simulink model "AnalysisSample11"  (R2021b)
settings: Solver=VariableStepAuto  StartTime=0.0  StopTime=10.0  RelTol=1e-3
settings Model: Creator=ygkwon  LastModifiedBy=ygkwon

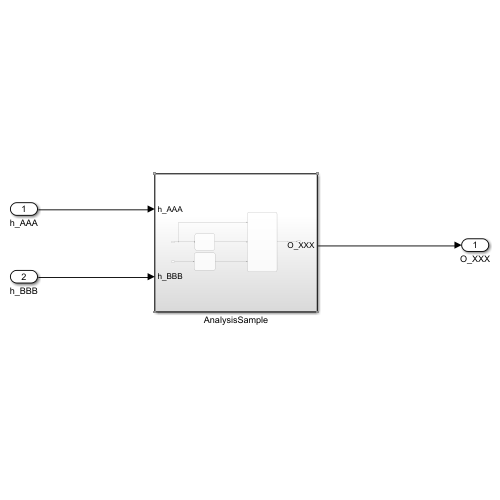
[thumbnail: Simulink's stored preview of the top-level diagram]
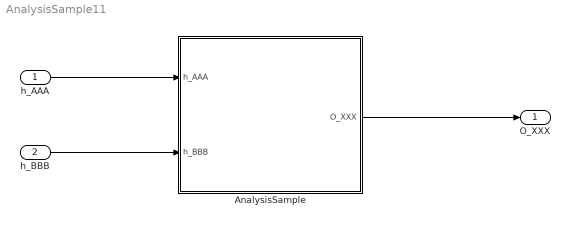
== system AnalysisSample11 ==
  h_AAA : Inport
  h_BBB : Inport  Port=2
  AnalysisSample : Subsystem
  O_XXX : Outport
  wires:
  h_AAA/1 -> AnalysisSample/1(h_AAA)
  AnalysisSample/1(O_XXX) -> O_XXX/1
  h_BBB/1 -> AnalysisSample/2(h_BBB)

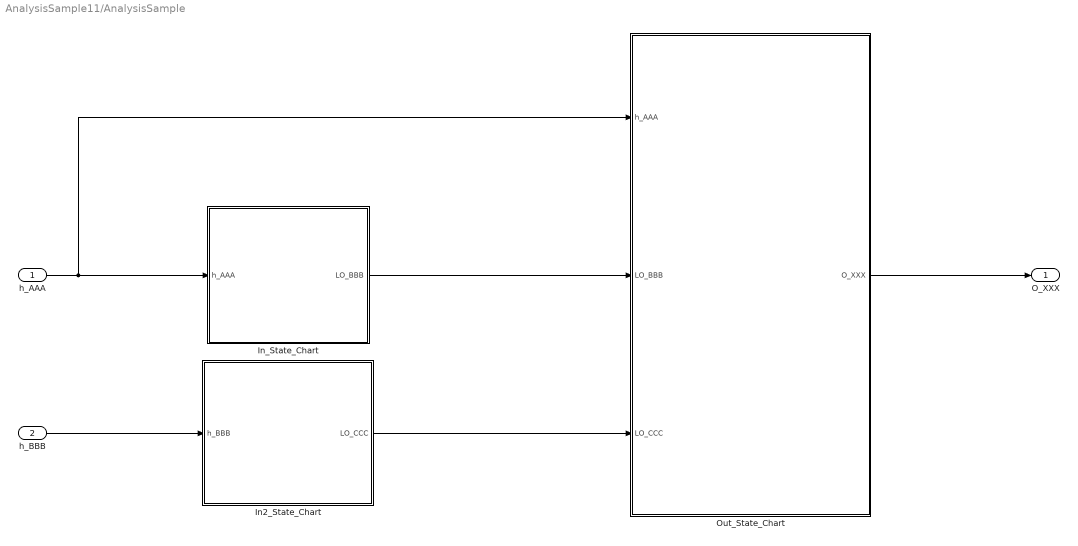
== system AnalysisSample11/AnalysisSample ==
  h_AAA : Inport
  h_BBB : Inport  Port=2
  In2_State_Chart : Stateflow chart  TreatAsAtomicUnit=on
  In_State_Chart : Stateflow chart  TreatAsAtomicUnit=on
  Out_State_Chart : Stateflow chart  TreatAsAtomicUnit=on
  O_XXX : Outport
  wires:
  In_State_Chart/1(LO_BBB) -> Out_State_Chart/2(LO_BBB)
  h_AAA/1 -> Out_State_Chart/1(h_AAA), In_State_Chart/1(h_AAA)
  Out_State_Chart/1(O_XXX) -> O_XXX/1
  h_BBB/1 -> In2_State_Chart/1(h_BBB)
  In2_State_Chart/1(LO_CCC) -> Out_State_Chart/3(LO_CCC)

== stateflow chart AnalysisSample11/AnalysisSample/In_State_Chart ==
  state Sample_State_Chart_2222
    en:
    LO_BBB = 22;
    state a
      en:
      LO_BBB=1;
    state a1
      en:
      LO_BBB=2;
    state a2
      en:
      LO_BBB=1;
    state a3
      en:
      LO_BBB=2;
      du:
      hello();
    (default) -> a [order 1] : [h_AAA == 11]
    a1 -> a [order 1] : [h_AAA==1]
    a1 -> a [order 2] : [h_AAA==11]
    a -> a1 : [h_AAA==2]
    (default) -> a2 [order 2]
    a3 -> a2 [order 1] : [h_AAA==1]
        | %hello
    a3 -> a2 [order 2] : [h_AAA==11]
    a2 -> a3 : [h_AAA==2]
  state hello [function]
    (default) -> (junction 20)
    (junction 20) -> (junction 24) [order 1] : [h_AAA == 111]
    (junction 20) -> (junction 22) [order 2]
    (junction 24) -> (junction 26) : {LO_BBB = 333;}
    (junction 26) -> (junction 22)
    (junction 22) -> (junction 29)
  data: h_AAA input uint8; LO_BBB output uint8

== stateflow chart AnalysisSample11/AnalysisSample/In2_State_Chart ==
  state Sample_State_Chart_3
    state b2
      en:
      LO_CCC=1;
    state b3
      en:
      LO_CCC=2;
    state a4
      en:
      LO_CCC=1;
    state a5
      en:
      LO_CCC=2;
    (default) -> b2 [order 1] : [h_BBB == 11]
    b3 -> b2 [order 1] : [h_BBB==1]
    b3 -> b2 [order 2] : [h_BBB==11]
    b2 -> b3 : [h_BBB==2]
    (default) -> a4 [order 2]
    a5 -> a4 [order 1] : [h_BBB==1]
        | %hello
    a5 -> a4 [order 2] : [h_BBB==11]
    a4 -> a5 : [h_BBB==2]
  data: h_BBB input; LO_CCC output double

== stateflow chart AnalysisSample11/AnalysisSample/Out_State_Chart ==
  state Sample_State_Chart_2222
    state a
      en:
      O_XXX=1;
    state a1
      en:
      O_XXX=2;
    state a2
      en:
      O_XXX=1;
    state a3
      en:
      O_XXX=2;
      du:
      hello();
    (default) -> a [order 1] : [h_AAA == 11]
    a1 -> a [order 1] : [h_AAA==11]
    a1 -> a [order 2] : [h_AAA==11]
    a -> a1 : [h_AAA==2]
    (default) -> a2 [order 2]
    a3 -> a2 [order 1] : [h_AAA==1]
        | %hello
    a3 -> a2 [order 2] : [h_AAA==11]
    a2 -> a3 : [h_AAA==2]
  state hello [function]
    (default) -> (junction 20)
    (junction 20) -> (junction 24) [order 1] : [h_AAA == 111&&...
        | LO_CCC==1]
    (junction 20) -> (junction 22) [order 2]
    (junction 24) -> (junction 26) : {O_XXX = 333;}
    (junction 26) -> (junction 22)
    (junction 22) -> (junction 29)
  data: h_AAA input uint8; LO_BBB input uint8; O_XXX output uint8; LO_CCC input uint8
